simulink model "duffing_cbc"  (R2023a)
settings: Solver=ode4  StartTime=0.0  StopTime=20  FixedStep=DeltaT  RelTol=1e-3
libraries: simulink x2
settings Model: Creator=akb110  LastModifiedBy=dionl
settings DataIOCC: LimitDataPoints=on  ReturnWorkspaceOutputs=off
settings OptimizationCC: OptimizeBlockIOStorage=off

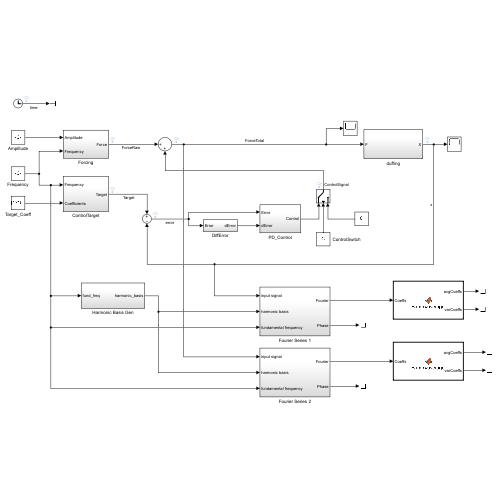
[thumbnail: Simulink's stored preview of the top-level diagram]
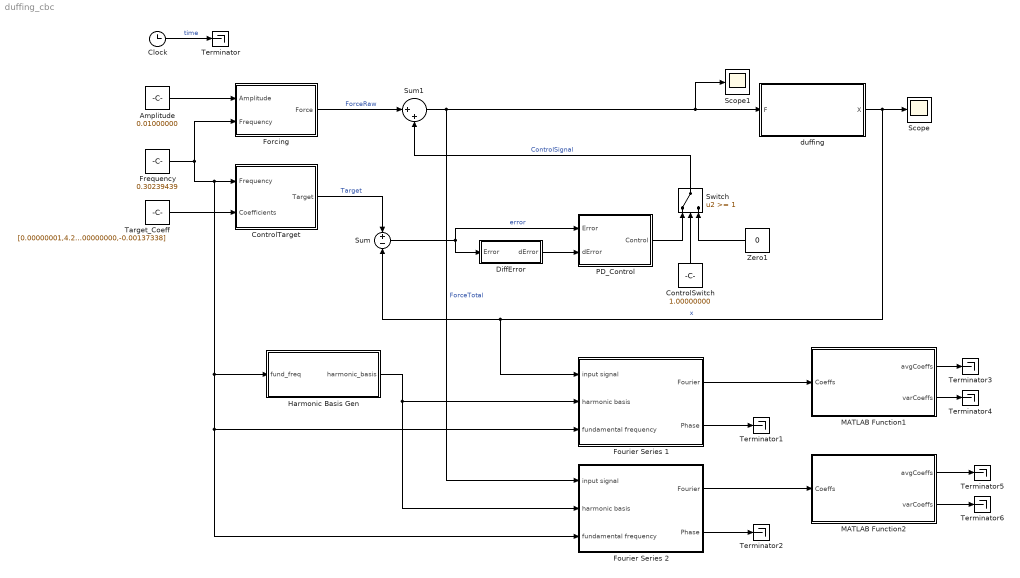
== system duffing_cbc ==
  Amplitude : Constant  Value=0.01000000
  Clock : Clock
  ControlSwitch : Constant  Value=1.00000000
  ControlTarget : Subsystem
  DiffError : Subsystem
  Forcing : Subsystem
  Fourier Series 1 : Subsystem
  Fourier Series 2 : Subsystem
  Frequency : Constant  Value=0.30239439
  Harmonic Basis Gen : Subsystem
  MATLAB Function1 : MATLAB Function  TreatAsAtomicUnit=on
  MATLAB Function2 : MATLAB Function  TreatAsAtomicUnit=on
  PD_Control : Subsystem
  Scope : Scope
  Scope1 : Scope
  Sum : Sum  Inputs=+|-
  Sum1 : Sum  Inputs=|++
  Switch : Switch  Threshold=1  SaturateOnIntegerOverflow=off  InputSameDT=off
  Target_Coeff : Constant  Value=[0.00000001,4.20000000,0.00000003,0.19283868,0.00000003,0.00963342,0.00000002,0.00022545,0.00000000,0.00000003,-0.13383079,0.00000001,-0.01518122,0.00000000,-0.00137338]
  Terminator{,1..6} (7 alike) : Terminator
  Zero1 : Constant  Value=0
  duffing : Subsystem
  wires:
  Frequency/1 -> Fourier Series 2/3(fundamental frequency), Fourier Series 1/3(fundamental frequency), Harmonic Basis Gen/1(fund_freq), ControlTarget/1(Frequency), Forcing/2(Frequency)
  Target_Coeff/1 -> ControlTarget/2(Coefficients)
  Amplitude/1 -> Forcing/1(Amplitude)
  ControlTarget/1(Target) -> Sum/1  "Target"
  duffing/1(X) -> Scope/1, Fourier Series 1/1(input signal), Sum/2  "x"
  Sum/1 -> PD_Control/1(Error), DiffError/1(Error)  "error"
  Switch/1 -> Sum1/2  "ControlSignal"
  DiffError/1(dError) -> PD_Control/2(dError)
  Zero1/1 -> Switch/3
  PD_Control/1(Control) -> Switch/1
  ControlSwitch/1 -> Switch/2
  Forcing/1(Force) -> Sum1/1  "ForceRaw"
  Sum1/1 -> Fourier Series 2/1(input signal), duffing/1(F), Scope1/1  "ForceTotal"
  Clock/1 -> Terminator/1  "time"
  Harmonic Basis Gen/1(harmonic_basis) -> Fourier Series 1/2(harmonic basis), Fourier Series 2/2(harmonic basis)
  Fourier Series 1/2(Phase) -> Terminator1/1
  Fourier Series 2/2(Phase) -> Terminator2/1
  Fourier Series 1/1(Fourier) -> MATLAB Function1/1(Coeffs)
  Fourier Series 2/1(Fourier) -> MATLAB Function2/1(Coeffs)
  MATLAB Function1/1(avgCoeffs) -> Terminator3/1
  MATLAB Function1/2(varCoeffs) -> Terminator4/1
  MATLAB Function2/1(avgCoeffs) -> Terminator5/1
  MATLAB Function2/2(varCoeffs) -> Terminator6/1

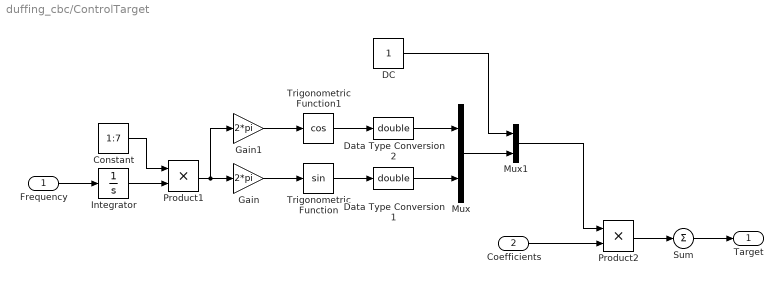
== system duffing_cbc/ControlTarget ==
  Frequency : Inport
  Coefficients : Inport  Port=2
  Constant : Constant  Value=1:7
  DC : Constant
  Data Type Conversion1 : DataTypeConversion  OutDataTypeStr=double  SaturateOnIntegerOverflow=off  RndMeth=Floor
  Data Type Conversion2 : DataTypeConversion  OutDataTypeStr=double  SaturateOnIntegerOverflow=off  RndMeth=Floor
  Gain : Gain  Gain=2*pi
  Gain1 : Gain  Gain=2*pi
  Integrator : Integrator
  Mux : Mux  Inputs=2
  Mux1 : Mux  Inputs=2
  Product1 : Product
  Product2 : Product  RndMeth=Zero
  Sum : Sum  Inputs=|+|
  Trigonometric Function : Trigonometry
  Trigonometric Function1 : Trigonometry  Operator=cos
  Target : Outport
  wires:
  Gain/1 -> Trigonometric Function/1
  Product2/1 -> Sum/1
  Gain1/1 -> Trigonometric Function1/1
  Sum/1 -> Target/1
  Frequency/1 -> Integrator/1
  Integrator/1 -> Product1/2
  Constant/1 -> Product1/1
  Trigonometric Function/1 -> Data Type Conversion1/1
  Mux1/1 -> Product2/1
  Trigonometric Function1/1 -> Data Type Conversion2/1
  Product1/1 -> Gain1/1, Gain/1
  Coefficients/1 -> Product2/2
  Data Type Conversion2/1 -> Mux/1
  Data Type Conversion1/1 -> Mux/2
  Mux/1 -> Mux1/2
  DC/1 -> Mux1/1

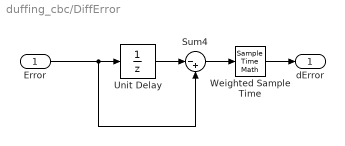
== system duffing_cbc/DiffError ==
  Error : Inport
  Sum4 : Sum  Inputs=|-+
  Unit Delay : UnitDelay  SampleTime=-1  HasFrameUpgradeWarning=on
  Weighted Sample Time : SampleTimeMath  TsampMathOp=/
  dError : Outport
  wires:
  Unit Delay/1 -> Sum4/1
  Sum4/1 -> Weighted Sample Time/1
  Weighted Sample Time/1 -> dError/1
  Error/1 -> Unit Delay/1, Sum4/2

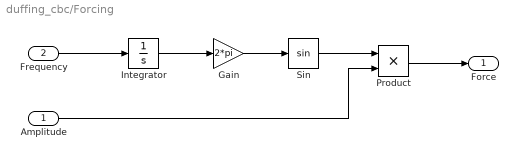
== system duffing_cbc/Forcing ==
  Amplitude : Inport
  Frequency : Inport  Port=2
  Gain : Gain  Gain=2*pi
  Integrator : Integrator
  Product : Product
  Sin : Trigonometry
  Force : Outport
  wires:
  Frequency/1 -> Integrator/1
  Gain/1 -> Sin/1
  Amplitude/1 -> Product/2
  Integrator/1 -> Gain/1
  Sin/1 -> Product/1
  Product/1 -> Force/1

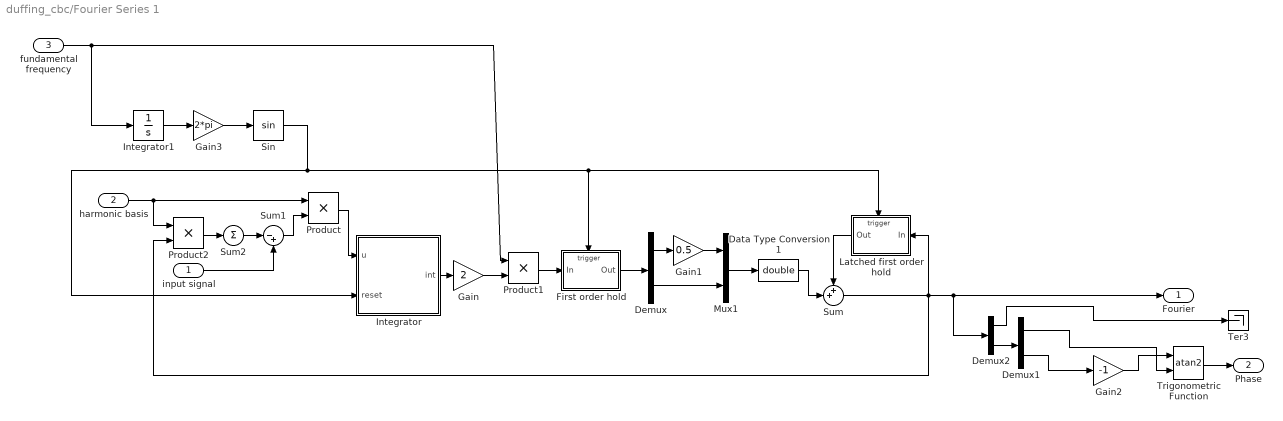
== system duffing_cbc/Fourier Series 1 ==
  input signal : Inport
  harmonic basis : Inport  Port=2
  fundamental frequency : Inport  Port=3
  Data Type Conversion1 : DataTypeConversion  OutDataTypeStr=double  SaturateOnIntegerOverflow=off  RndMeth=Floor
  Demux : Demux  Outputs=[1 -1]
  Demux1 : Demux  Outputs=2
  Demux2 : Demux  Outputs=[1 -1]
  First order hold : Subsystem  TreatAsAtomicUnit=on
  Gain : Gain  Gain=2
  Gain1 : Gain  Gain=0.5
  Gain2 : Gain  Gain=-1
  Gain3 : Gain  Gain=2*pi
  Integrator : Subsystem
  Integrator1 : Integrator
  Latched first order hold : Subsystem  TreatAsAtomicUnit=on
  Mux1 : Mux  Inputs=2
  Product : Product  RndMeth=Zero
  Product1 : Product  RndMeth=Zero
  Product2 : Product  RndMeth=Zero
  Sin : Trigonometry
  Sum : Sum  Tag=Test  Inputs=++|
  Sum1 : Sum  Inputs=|-+
  Sum2 : Sum  Inputs=|+|
  Ter3 : Terminator
  Trigonometric Function : Trigonometry  Operator=atan2
  Fourier : Outport
  Phase : Outport  Port=2
  wires:
  Product1/1 -> First order hold/1(In)
  Gain/1 -> Product1/2
  Sin/1 -> Integrator/2(reset), First order hold/Trigger, Latched first order hold/Trigger
  Integrator/1(int) -> Gain/1
  Demux/1 -> Gain1/1
  Gain1/1 -> Mux1/1
  Demux/2 -> Mux1/2
  First order hold/1(Out) -> Demux/1
  Mux1/1 -> Data Type Conversion1/1
  Data Type Conversion1/1 -> Sum/2
  Sum/1 -> Product2/2, Latched first order hold/1(In), Fourier/1, Demux2/1
  Latched first order hold/1(Out) -> Sum/1
  Sum1/1 -> Product/2
  Product2/1 -> Sum2/1
  input signal/1 -> Sum1/2
  harmonic basis/1 -> Product/1, Product2/1
  Sum2/1 -> Sum1/1
  Trigonometric Function/1 -> Phase/1
  Product/1 -> Integrator/1(u)
  Demux1/1 -> Trigonometric Function/2
  Demux1/2 -> Gain2/1
  Gain2/1 -> Trigonometric Function/1
  Demux2/2 -> Demux1/1
  Demux2/1 -> Ter3/1
  Gain3/1 -> Sin/1
  Integrator1/1 -> Gain3/1
  fundamental frequency/1 -> Integrator1/1, Product1/1

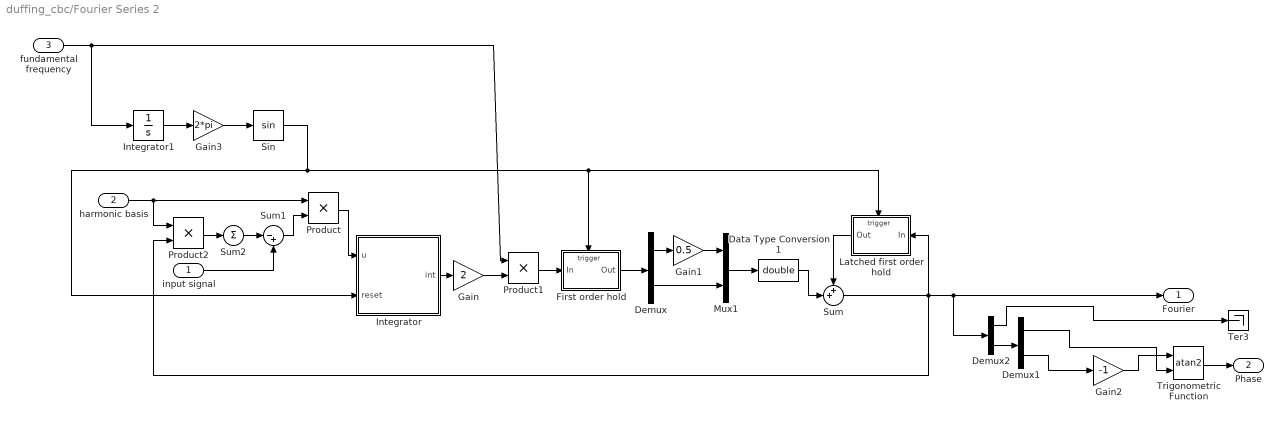
== system duffing_cbc/Fourier Series 2 ==
  input signal : Inport
  harmonic basis : Inport  Port=2
  fundamental frequency : Inport  Port=3
  Data Type Conversion1 : DataTypeConversion  OutDataTypeStr=double  SaturateOnIntegerOverflow=off  RndMeth=Floor
  Demux : Demux  Outputs=[1 -1]
  Demux1 : Demux  Outputs=2
  Demux2 : Demux  Outputs=[1 -1]
  First order hold : Subsystem  TreatAsAtomicUnit=on
  Gain : Gain  Gain=2
  Gain1 : Gain  Gain=0.5
  Gain2 : Gain  Gain=-1
  Gain3 : Gain  Gain=2*pi
  Integrator : Subsystem
  Integrator1 : Integrator
  Latched first order hold : Subsystem  TreatAsAtomicUnit=on
  Mux1 : Mux  Inputs=2
  Product : Product  RndMeth=Zero
  Product1 : Product  RndMeth=Zero
  Product2 : Product  RndMeth=Zero
  Sin : Trigonometry
  Sum : Sum  Tag=Test  Inputs=++|
  Sum1 : Sum  Inputs=|-+
  Sum2 : Sum  Inputs=|+|
  Ter3 : Terminator
  Trigonometric Function : Trigonometry  Operator=atan2
  Fourier : Outport
  Phase : Outport  Port=2
  wires:
  Product1/1 -> First order hold/1(In)
  Gain/1 -> Product1/2
  Sin/1 -> Integrator/2(reset), First order hold/Trigger, Latched first order hold/Trigger
  Integrator/1(int) -> Gain/1
  Demux/1 -> Gain1/1
  Gain1/1 -> Mux1/1
  Demux/2 -> Mux1/2
  First order hold/1(Out) -> Demux/1
  Mux1/1 -> Data Type Conversion1/1
  Data Type Conversion1/1 -> Sum/2
  Sum/1 -> Product2/2, Latched first order hold/1(In), Fourier/1, Demux2/1
  Latched first order hold/1(Out) -> Sum/1
  Sum1/1 -> Product/2
  Product2/1 -> Sum2/1
  input signal/1 -> Sum1/2
  harmonic basis/1 -> Product/1, Product2/1
  Sum2/1 -> Sum1/1
  Trigonometric Function/1 -> Phase/1
  Product/1 -> Integrator/1(u)
  Demux1/1 -> Trigonometric Function/2
  Demux1/2 -> Gain2/1
  Gain2/1 -> Trigonometric Function/1
  Demux2/2 -> Demux1/1
  Demux2/1 -> Ter3/1
  Gain3/1 -> Sin/1
  Integrator1/1 -> Gain3/1
  fundamental frequency/1 -> Integrator1/1, Product1/1

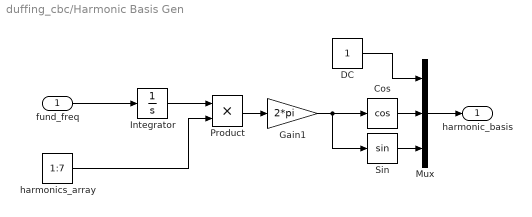
== system duffing_cbc/Harmonic Basis Gen ==
  fund_freq : Inport
  Cos : Trigonometry  Operator=cos
  DC : Constant
  Gain1 : Gain  Gain=2*pi
  Integrator : Integrator
  Mux : Mux  Inputs=3
  Product : Product
  Sin : Trigonometry
  harmonics_array : Constant  Value=1:7
  harmonic_basis : Outport  OutDataTypeStr=double  SampleTime=0
  wires:
  Gain1/1 -> Sin/1, Cos/1
  Mux/1 -> harmonic_basis/1
  Integrator/1 -> Product/1
  Cos/1 -> Mux/2
  Product/1 -> Gain1/1
  Sin/1 -> Mux/3
  harmonics_array/1 -> Product/2
  fund_freq/1 -> Integrator/1
  DC/1 -> Mux/1

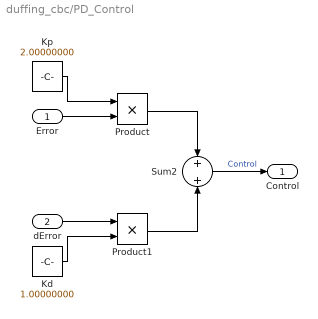
== system duffing_cbc/PD_Control ==
  Error : Inport
  dError : Inport  Port=2
  Kd : Constant  Value=1.00000000
  Kp : Constant  Value=2.00000000
  Product : Product  RndMeth=Zero
  Product1 : Product  RndMeth=Zero
  Sum2 : Sum  Inputs=+|+
  Control : Outport
  wires:
  Kp/1 -> Product/1
  Kd/1 -> Product1/2
  Product/1 -> Sum2/1
  Product1/1 -> Sum2/2
  Error/1 -> Product/2
  Sum2/1 -> Control/1  "Control"
  dError/1 -> Product1/1

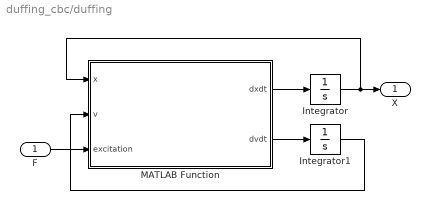
== system duffing_cbc/duffing ==
  F : Inport
  Integrator : Integrator
  Integrator1 : Integrator
  MATLAB Function : MATLAB Function  TreatAsAtomicUnit=on
  X : Outport
  wires:
  Integrator1/1 -> MATLAB Function/2(v)
  MATLAB Function/2(dvdt) -> Integrator1/1
  MATLAB Function/1(dxdt) -> Integrator/1
  F/1 -> MATLAB Function/3(excitation)
  Integrator/1 -> MATLAB Function/1(x), X/1

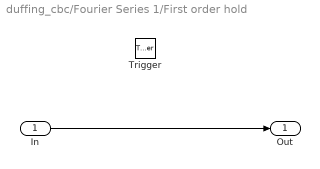
== system duffing_cbc/Fourier Series 1/First order hold ==
  In : Inport  LatchByDelayingOutsideSignal=on
  Trigger : TriggerPort  VariantControl=(inherit)
  Out : Outport
  wires:
  In/1 -> Out/1

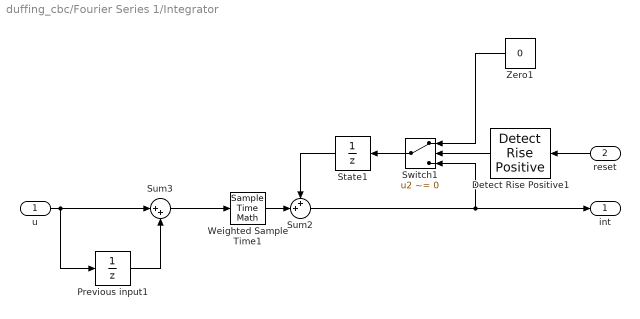
== system duffing_cbc/Fourier Series 1/Integrator ==
  u : Inport
  reset : Inport  Port=2
  Detect Rise Positive1 : simulink/Logic and Bit Operations/Detect Rise Positive  vinit=0  OutDataTypeStr=uint8
  Previous input1 : UnitDelay  SampleTime=-1  HasFrameUpgradeWarning=on
  State1 : UnitDelay  SampleTime=-1  HasFrameUpgradeWarning=on
  Sum2 : Sum  Inputs=++|
  Sum3 : Sum  Inputs=|++
  Switch1 : Switch  Criteria=u2 ~= 0  SaturateOnIntegerOverflow=off  InputSameDT=off
  Weighted Sample Time1 : SampleTimeMath  TsampMathOp=*  weightValue=0.5
  Zero1 : Constant  Value=0
  int : Outport
  wires:
  Detect Rise Positive1/1 -> Switch1/2
  Zero1/1 -> Switch1/1
  Switch1/1 -> State1/1
  reset/1 -> Detect Rise Positive1/1
  Previous input1/1 -> Sum3/2
  u/1 -> Previous input1/1, Sum3/1
  Sum3/1 -> Weighted Sample Time1/1
  Weighted Sample Time1/1 -> Sum2/2
  Sum2/1 -> int/1, Switch1/3
  State1/1 -> Sum2/1

== system duffing_cbc/Fourier Series 1/Latched first order hold ==
  In : Inport  LatchByDelayingOutsideSignal=on
  Trigger : TriggerPort  VariantControl=(inherit)
  Out : Outport
  wires:
  In/1 -> Out/1

== system duffing_cbc/Fourier Series 2/First order hold ==
  In : Inport  LatchByDelayingOutsideSignal=on
  Trigger : TriggerPort  VariantControl=(inherit)
  Out : Outport
  wires:
  In/1 -> Out/1

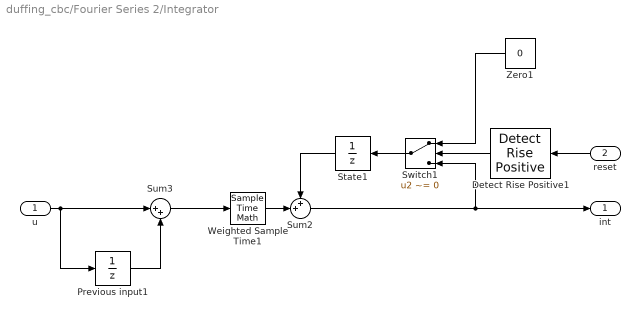
== system duffing_cbc/Fourier Series 2/Integrator ==
  u : Inport
  reset : Inport  Port=2
  Detect Rise Positive1 : simulink/Logic and Bit Operations/Detect Rise Positive  vinit=0  OutDataTypeStr=uint8
  Previous input1 : UnitDelay  SampleTime=-1  HasFrameUpgradeWarning=on
  State1 : UnitDelay  SampleTime=-1  HasFrameUpgradeWarning=on
  Sum2 : Sum  Inputs=++|
  Sum3 : Sum  Inputs=|++
  Switch1 : Switch  Criteria=u2 ~= 0  SaturateOnIntegerOverflow=off  InputSameDT=off
  Weighted Sample Time1 : SampleTimeMath  TsampMathOp=*  weightValue=0.5
  Zero1 : Constant  Value=0
  int : Outport
  wires:
  Detect Rise Positive1/1 -> Switch1/2
  Zero1/1 -> Switch1/1
  Switch1/1 -> State1/1
  reset/1 -> Detect Rise Positive1/1
  Previous input1/1 -> Sum3/2
  u/1 -> Previous input1/1, Sum3/1
  Sum3/1 -> Weighted Sample Time1/1
  Weighted Sample Time1/1 -> Sum2/2
  Sum2/1 -> int/1, Switch1/3
  State1/1 -> Sum2/1

== system duffing_cbc/Fourier Series 2/Latched first order hold ==
  In : Inport  LatchByDelayingOutsideSignal=on
  Trigger : TriggerPort  VariantControl=(inherit)
  Out : Outport
  wires:
  In/1 -> Out/1

== matlab function duffing_cbc/MATLAB Function1 ==
  data: Coeffs input; avgCoeffs output double size=30; varCoeffs output size=30
function [avgCoeffs, varCoeffs] = windowaverage(Coeffs)
% movingFourierStats computes a moving average and variance of Fourier coefficients
% over a given number of samples
%
% Inputs:
%   fourierCoeffs - Fourier coefficients vector
%
% Outputs:
%   avgCoeffs     - Moving average of the Fourier coefficients
%   varCoeffs     - Moving variance
%

% Number of samples for averaging
Nwindow = 10;

% Initialize persistent variables.
persistent buffer idx count numCoeffs
if isempty(buffer)
    numCoeffs = length(Coeffs);
    buffer = zeros(Nwindow, numCoeffs);  % Preallocate circular buffer.
    idx = 1;      % Current insertion index.
    count = 0;    % Number of valid samples stored.
end

sample = Coeffs(:).';

% Insert the new sample into the circular buffer.
buffer(idx, :) = sample;

% Update the circular buffer index.
idx = idx + 1;
if idx > Nwindow
    idx = 1;
end

% Increase the count until the buffer is full.
if count < Nwindow
    count = count + 1;
end

% Compute the moving average across the stored samples.
avgRow = mean(buffer(1:count, :), 1);
avgCoeffs = avgRow.';

% Compute the moving variance for each coefficient.
varRow = sum((buffer(1:count, :) - repmat(avgRow, count, 1)).^2, 1) / count;
varCoeffs = varRow.';

end

== matlab function duffing_cbc/duffing/MATLAB Function ==
  data: x input; dxdt output; v input; excitation input; dvdt output
function [dxdt, dvdt] = duffingDerivatives(x, v, excitation)
% Duffing oscillator derivatives
%
% Inputs:
%   x - displacement
%   v - velocity
%   excitation - external excitation signal
%
% Outputs:
%   dx/dt dv/dt

% Define Duffing parameters

% stable duffing
% delta = 0.2;    % damping
% alpha = +1;     % linear stiffness
% beta  = 1;      % nonlinear stiffness

% bi-stable duffing
delta = 0.2;    % damping
alpha = -1;     % linear stiffness
beta  = 1;      % nonlinear stiffness

% bi-stable duffing from Rezaee, Renson: https://doi.org/10.1137/23M1587774
% delta = 0.1;    % damping
% alpha = -4;     % linear stiffness
% beta  = 2;      % nonlinear stiffness


% Duffing equation derivatives
dxdt = v;
dvdt = excitation - delta*v - alpha*x - beta*x^3;

end

== matlab function duffing_cbc/MATLAB Function2 ==
  data: Coeffs input; avgCoeffs output double size=30; varCoeffs output size=30
function [avgCoeffs, varCoeffs] = windowaverage(Coeffs)
% movingFourierStats computes a moving average and variance of Fourier coefficients
% over a given number of samples
%
% Inputs:
%   fourierCoeffs - Fourier coefficients vector
%
% Outputs:
%   avgCoeffs     - Moving average of the Fourier coefficients
%   varCoeffs     - Moving variance
%

% Number of samples for averaging
Nwindow = 10;

% Initialize persistent variables.
persistent buffer idx count numCoeffs
if isempty(buffer)
    numCoeffs = length(Coeffs);
    buffer = zeros(Nwindow, numCoeffs);  % Preallocate circular buffer.
    idx = 1;      % Current insertion index.
    count = 0;    % Number of valid samples stored.
end

sample = Coeffs(:).';

% Insert the new sample into the circular buffer.
buffer(idx, :) = sample;

% Update the circular buffer index.
idx = idx + 1;
if idx > Nwindow
    idx = 1;
end

% Increase the count until the buffer is full.
if count < Nwindow
    count = count + 1;
end

% Compute the moving average across the stored samples.
avgRow = mean(buffer(1:count, :), 1);
avgCoeffs = avgRow.';

% Compute the moving variance for each coefficient.
varRow = sum((buffer(1:count, :) - repmat(avgRow, count, 1)).^2, 1) / count;
varCoeffs = varRow.';

end
